simulink model "untitled"  (R2015a)
settings: Solver=ode45  StartTime=0.0  StopTime=30  FixedStep=10e-3  RelTol=1e-3
values from neighbouring files (symbols this model uses):
  A1 = (m1*g+k*l1)/l1/m1    (= 2.962)    [Parametri.m]
  A2 = k*l2/l1/m1    (= 1)    [Parametri.m]
  A3 = (m2*g+k*l2)/l2/m2    (= 2.962)    [Parametri.m]
  A4 = k*l1/l2/m2    (= 1)    [Parametri.m]
  l1 = 5    [Parametri.m]
  l2 = 5    [Parametri.m]
  teta1 = 0.5    [Parametri.m]
  teta2 = 0.5    [Parametri.m]
  v1 = 0    [Parametri.m]
  v2 = -0    (= 0)    [Parametri.m]
libraries: dspspect3 x1, dspxfrm3 x1
settings Model: Creator=BLAGI  LastModifiedBy=BLAGI

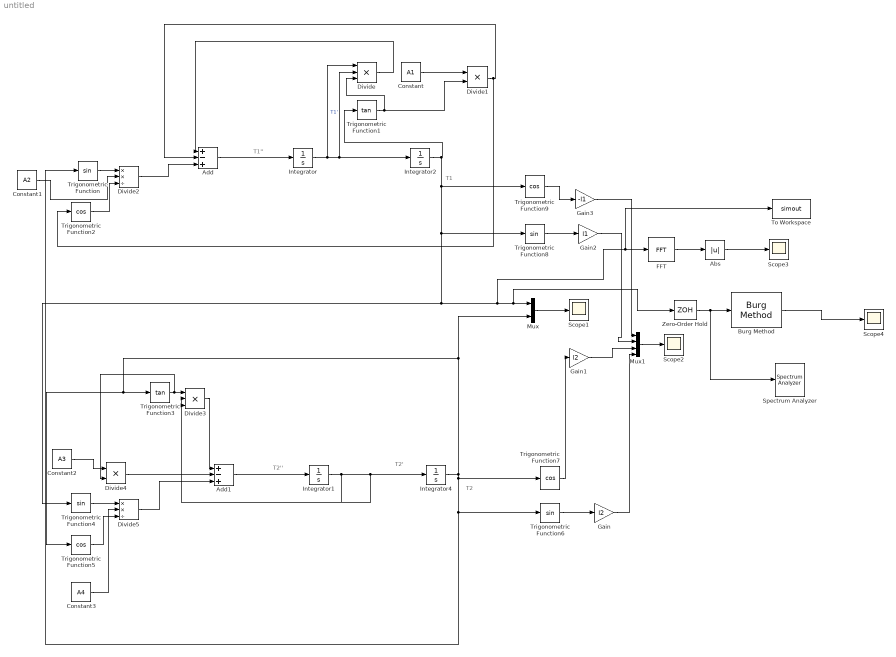
== system untitled ==
  note: T2
  note: T1
  note: T1''
  note: T2'
  note: T2''
  Abs : Abs
  Add : Sum  Inputs=+-+
  Add1 : Sum  Inputs=+-+
  Burg Method : dspspect3/Burg Method  inheritOrd=on  ord=6  inheritFFT=on  fftsize=2560  inheritTs=on  Ts=1
  Constant : Constant  Value=A1
  Constant1 : Constant  Value=A2
  Constant2 : Constant  Value=A3
  Constant3 : Constant  Value=A4
  Divide : Product  Inputs=***
  Divide1 : Product  Inputs=**
  Divide2 : Product  Inputs=**/
  Divide3 : Product  Inputs=***
  Divide4 : Product  Inputs=**
  Divide5 : Product  Inputs=**/
  FFT : dspxfrm3/FFT  CompMethod=Table lookup  TableOpt=NEW  TableOptActive=Speed  BitRevOrder=off  InheritFFTLength=on  FFTLength=64  WrapInput=on  RowConvenienceOn=on  FFTImplementation=Auto  SkipNorm=off  firstCoeffDataTypeStr=Inherit: Same word length as input  firstCoeffLastDataTypeStr=Inherit: Same word length as input  outputMin=[]  outputMax=[]  roundingMode=Floor  overflowMode=off
  Gain : Gain  Gain=l2
  Gain1 : Gain  Gain=l2
  Gain2 : Gain  Gain=l1
  Gain3 : Gain  Gain=-l1
  Integrator : Integrator  InitialCondition=v1  LimitOutput=on  UpperSaturationLimit=14  LowerSaturationLimit=-14
  Integrator1 : Integrator  InitialCondition=v2  LimitOutput=on  UpperSaturationLimit=14  LowerSaturationLimit=-14
  Integrator2 : Integrator  InitialCondition=teta1  LimitOutput=on  UpperSaturationLimit=45  LowerSaturationLimit=-45
  Integrator4 : Integrator  InitialCondition=teta2  LimitOutput=on  UpperSaturationLimit=45  LowerSaturationLimit=-45
  Mux : Mux  Inputs=2
  Mux1 : Mux
  Scope{1..4} (4 alike) : Scope
      Scope3 settings: SaveName=ScopeData2
      Scope4 settings: YMin=-1  YMax=1.5  SaveName=ScopeData3
  Spectrum Analyzer : SpectrumAnalyzer
  To Workspace : ToWorkspace  VariableName=simout  SampleTime=-1
  Trigonometric Function{,4,6,8} (4 alike) : Trigonometry
  Trigonometric Function1 : Trigonometry  Operator=tan
  Trigonometric Function{2,5,7,9} (4 alike) : Trigonometry  Operator=cos
  Trigonometric Function3 : Trigonometry  Operator=tan
  Zero-Order Hold : ZeroOrderHold  SampleTime=0.01
  wires:
  Add/1 -> Integrator/1
  Integrator/1 -> Divide/1, Divide/2, Integrator2/1  "T1'"
  Add1/1 -> Integrator1/1
  Trigonometric Function1/1 -> Divide1/2, Divide/3
  Divide/1 -> Add/1
  Constant/1 -> Divide1/1
  Divide1/1 -> Trigonometric Function2/1, Add/2
  Trigonometric Function/1 -> Divide2/1
  Trigonometric Function2/1 -> Divide2/3
  Constant1/1 -> Divide2/2
  Divide2/1 -> Add/3
  Trigonometric Function3/1 -> Divide4/2, Divide3/1
  Integrator1/1 -> Divide3/2, Integrator4/1, Divide3/3
  Divide3/1 -> Add1/1
  Constant2/1 -> Divide4/1
  Divide4/1 -> Add1/2
  Divide5/1 -> Add1/3
  Trigonometric Function4/1 -> Divide5/1
  Constant3/1 -> Divide5/2
  Trigonometric Function5/1 -> Divide5/3
  Mux/1 -> Scope1/1
  Trigonometric Function6/1 -> Gain/1
  Trigonometric Function7/1 -> Gain1/1
  Trigonometric Function8/1 -> Gain2/1
  Trigonometric Function9/1 -> Gain3/1
  Gain2/1 -> Mux1/2
  Mux1/1 -> Scope2/1
  Gain3/1 -> Mux1/1
  Gain/1 -> Mux1/4
  Gain1/1 -> Mux1/3
  Integrator4/1 -> Trigonometric Function7/1, Trigonometric Function6/1, Trigonometric Function/1, Mux/2, Trigonometric Function3/1, Trigonometric Function5/1
  Abs/1 -> Scope3/1
  FFT/1 -> Abs/1
  Burg Method/1 -> Scope4/1
  Zero-Order Hold/1 -> Spectrum Analyzer/1, Burg Method/1
  Integrator2/1 -> Trigonometric Function8/1, FFT/1, To Workspace/1, Zero-Order Hold/1, Mux/1, Trigonometric Function4/1, Trigonometric Function9/1, Trigonometric Function1/1
